simulink model "Load_torque_2nd_order_estimator"  (R2021a)
settings: Solver=FixedStepDiscrete  StartTime=0.0  StopTime=10.0  FixedStep=1e-05  MaxStep=1e-05  RelTol=1e-3
undefined symbols (not defined in the file): DiscIntNeverNeededParam
settings Model: Creator=Mehra  LastModifiedBy=Mehra

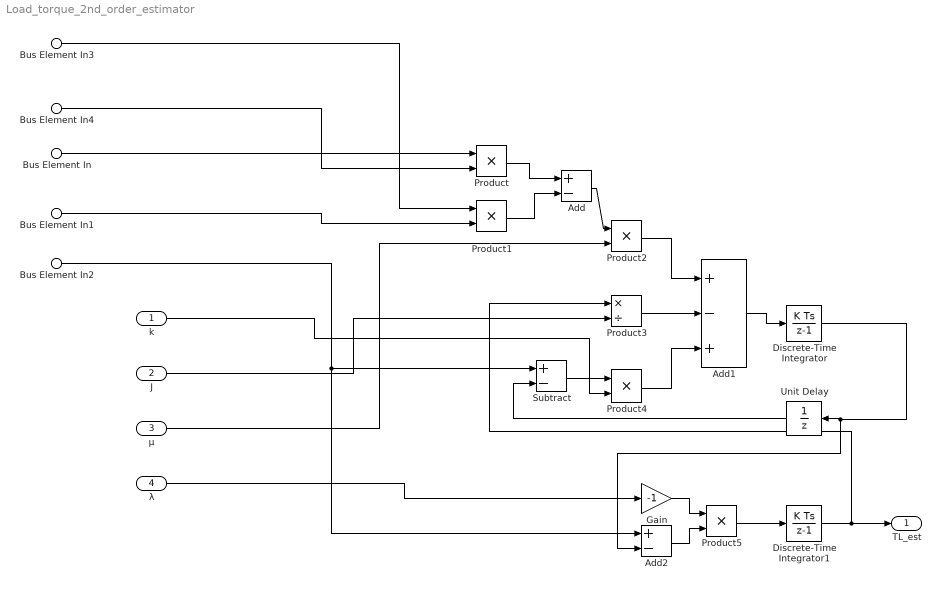
== system Load_torque_2nd_order_estimator ==
  k : Inport
  J : Inport  Port=2
  µ : Inport  Port=3
  λ : Inport  Port=4
  Bus Element In4 : Inport  Port=5  PortName=mesin  Element=Isb
  Bus Element In3 : Inport  Port=5  PortName=mesin  Element=Isa
  Bus Element In : Inport  Port=5  PortName=mesin  Element=Ψra
  Bus Element In1 : Inport  Port=5  PortName=mesin  Element=Ψrb
  Bus Element In2 : Inport  Port=5  PortName=mesin  Element=ω
  Add : Sum  Inputs=+-
  Add1 : Sum  Inputs=+-+
  Add2 : Sum  Inputs=+-
  Discrete-Time Integrator : DiscreteIntegrator  SampleTime=-1  ICPrevOutput=DiscIntNeverNeededParam  ICPrevScaledInput=DiscIntNeverNeededParam
  Discrete-Time Integrator1 : DiscreteIntegrator  SampleTime=-1  ICPrevOutput=DiscIntNeverNeededParam  ICPrevScaledInput=DiscIntNeverNeededParam
  Gain : Gain  Gain=-1
  Product{,1..2,4..5} (5 alike) : Product
  Product3 : Product  Inputs=*/
  Subtract : Sum  Inputs=+-
  Unit Delay : UnitDelay  SampleTime=-1  HasFrameUpgradeWarning=on
  TL_est : Outport
  wires:
  Product/1 -> Add/1
  Product1/1 -> Add/2
  Add/1 -> Product2/1
  µ/1 -> Product2/2
  J/1 -> Product3/2
  Subtract/1 -> Product4/1
  Bus Element In2/1 -> Add2/1, Subtract/1
  k/1 -> Product4/2
  Product2/1 -> Add1/1
  Product3/1 -> Add1/2
  Product4/1 -> Add1/3
  Add2/1 -> Product5/2
  Gain/1 -> Product5/1
  λ/1 -> Gain/1
  Add1/1 -> Discrete-Time Integrator/1
  Product5/1 -> Discrete-Time Integrator1/1
  Bus Element In/1 -> Product/1
  Bus Element In4/1 -> Product/2
  Bus Element In1/1 -> Product1/2
  Bus Element In3/1 -> Product1/1
  Discrete-Time Integrator/1 -> Unit Delay/1, Add2/2
  Discrete-Time Integrator1/1 -> Product3/1, TL_est/1
  Unit Delay/1 -> Subtract/2
